simulink model "AirPropsEx"  (R2015a)
settings: Solver=ode45  StartTime=0.0  StopTime=10.0  RelTol=1e-3
libraries: lib_AirProps_HeatCapacity x1, lib_AirProps_SpecificHeatConstVol x1, lib_AirProps_ThermCond x1, lib_AirProps_Viscosity x1
settings Model: Creator=jlkratz  LastModifiedBy=jlkratz

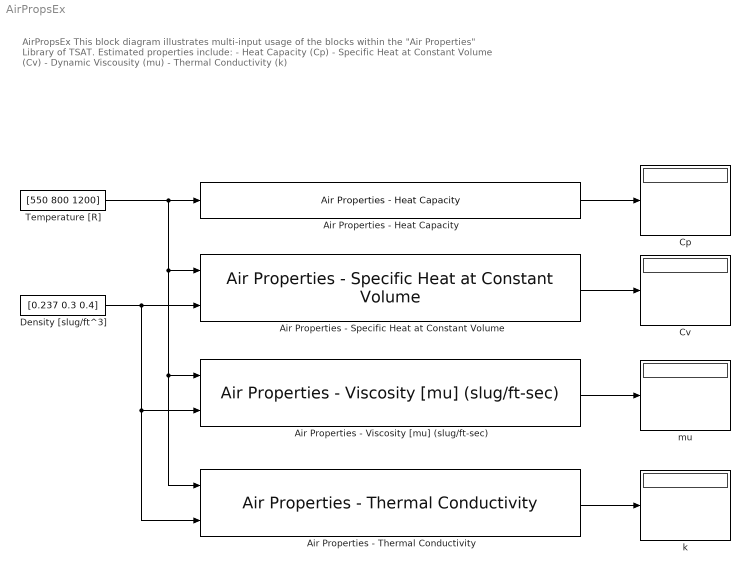
== system AirPropsEx ==
  note: AirPropsEx
      |
      | This block diagram illustrates multi-input usage of the blocks within the "Air Properties" Library of TSAT. Estimated properties include:
      | - Heat Capacity (Cp)
      | - Specific Heat at Constant Volume (Cv)
      | - Dynamic Viscousity (mu)
      | - Thermal Conductivity (k)
  Air Properties - Heat Capacity : lib_AirProps_HeatCapacity/Air Properties - Heat Capacity  BN_M=double(gcb)
  Air Properties - Specific Heat at Constant Volume : lib_AirProps_SpecificHeatConstVol/Air Properties - Specific Heat at Constant Volume  BN_M=double(gcb)
  Air Properties - Thermal Conductivity : lib_AirProps_ThermCond/Air Properties - Thermal Conductivity  BN_M=double(gcb)
  Air Properties - Viscosity [mu] (slug/ft-sec) : lib_AirProps_Viscosity/Air Properties - Viscosity [mu] (slug//ft-sec)  BN_M=double(gcb)
  Cp : Display
  Cv : Display
  Density [slug/ft^3] : Constant  Value=[0.237 0.3 0.4]
  Temperature [R] : Constant  Value=[550 800 1200]
  k : Display
  mu : Display
  wires:
  Density [slug/ft^3]/1 -> Air Properties - Thermal Conductivity/2, Air Properties - Viscosity [mu] (slug/ft-sec)/2, Air Properties - Specific Heat at Constant Volume/2
  Temperature [R]/1 -> Air Properties - Thermal Conductivity/1, Air Properties - Viscosity [mu] (slug/ft-sec)/1, Air Properties - Specific Heat at Constant Volume/1, Air Properties - Heat Capacity/1
  Air Properties - Heat Capacity/1 -> Cp/1
  Air Properties - Specific Heat at Constant Volume/1 -> Cv/1
  Air Properties - Viscosity [mu] (slug/ft-sec)/1 -> mu/1
  Air Properties - Thermal Conductivity/1 -> k/1
